simulink model "model_mussels"  (R2014b)
settings: Solver=ode45  StartTime=0.0  StopTime=40  MaxStep=0.01  RelTol=1e-3
undefined symbols (not defined in the file or in its folder): adapt, c, K, pos_0, sigma_0, speed, zeta_0
settings Model: CovSFcnEnable=on  Creator=Marta_2805  LastModifiedBy=Annie
settings SolverCC: AutoInsertRateTranBlk=on
settings OptimizationCC: UseDivisionForNetSlopeComputation=off  SimCompilerOptimization=off
settings DebuggingCC: UnderspecifiedInitializationDetection=Classic  MergeDetectMultiDrivingBlocksExec=none  FrameProcessingCompatibilityMsg=error
settings RTWCC: RTWCompilerOptimization=off

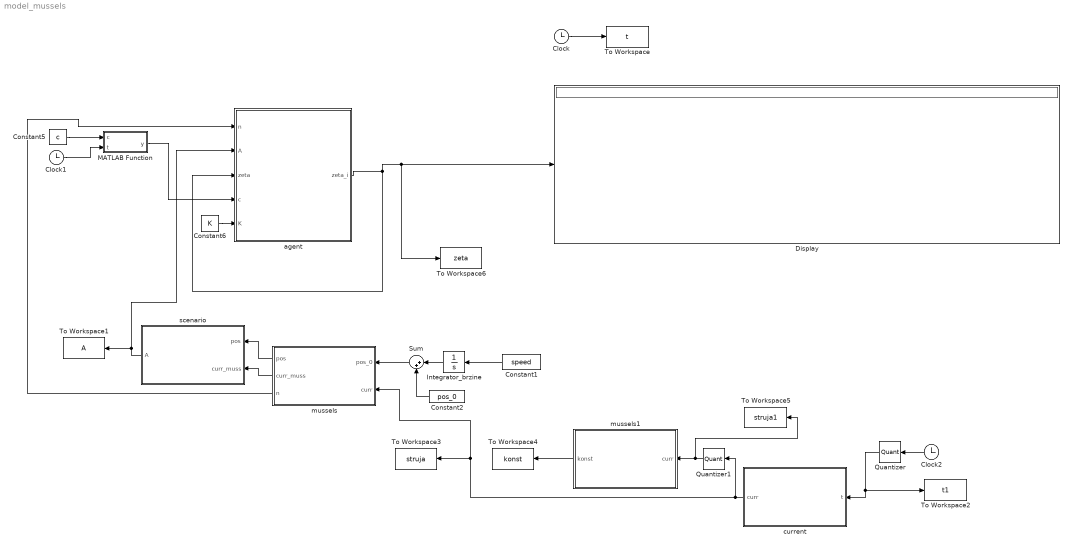
== system model_mussels ==
  Clock : Clock
  Clock1 : Clock
  Clock2 : Clock
      settings: Decimation=1000
  Constant1 : Constant  Value=speed
  Constant2 : Constant  Value=pos_0
  Constant5 : Constant  Value=c
  Constant6 : Constant  Value=K
  Display : Display
  Integrator_brzine : Integrator  InitialCondition=[0 0 0 0 0;0 0 0 0 0;0 0 0 0 0]
  MATLAB Function : MATLAB Function  TreatAsAtomicUnit=on
  Quantizer : Quantizer  QuantizationInterval=1
  Quantizer1 : Quantizer  QuantizationInterval=0.0001
  Sum : Sum  Inputs=|++
  To Workspace : ToWorkspace  VariableName=t  SampleTime=-1
  To Workspace1 : ToWorkspace  VariableName=A  SampleTime=-1
  To Workspace2 : ToWorkspace  VariableName=t1  SampleTime=-1
  To Workspace3 : ToWorkspace  VariableName=struja  SampleTime=-1
  To Workspace4 : ToWorkspace  VariableName=konst  SampleTime=-1
  To Workspace5 : ToWorkspace  VariableName=struja1  SampleTime=-1
  To Workspace6 : ToWorkspace  VariableName=zeta  SampleTime=-1
  "agent " : Subsystem
  current : MATLAB Function  TreatAsAtomicUnit=on
  mussels : MATLAB Function  TreatAsAtomicUnit=on
  mussels1 : MATLAB Function  TreatAsAtomicUnit=on
  scenario : MATLAB Function  TreatAsAtomicUnit=on
  wires:
  Constant6/1 -> "agent "/5(K)
  MATLAB Function/1(y) -> "agent "/4(c)
  "agent "/1(zeta_i) -> "agent "/3(zeta), Display/1, To Workspace6/1
  Constant5/1 -> MATLAB Function/1(c)
  Clock1/1 -> MATLAB Function/2(t)
  mussels/1(pos) -> scenario/1(pos)
  scenario/1(A) -> To Workspace1/1, "agent "/2(A)
  mussels/3(n) -> "agent "/1(n)
  Sum/1 -> mussels/1(pos_0)
  Clock/1 -> To Workspace/1
  Constant1/1 -> Integrator_brzine/1
  Constant2/1 -> Sum/2
  Integrator_brzine/1 -> Sum/1
  Clock2/1 -> Quantizer/1
  Quantizer/1 -> To Workspace2/1, current/1(t)
  current/1(curr) -> mussels/2(curr), To Workspace3/1, Quantizer1/1
  mussels/2(curr_muss) -> scenario/2(curr_muss)
  Quantizer1/1 -> mussels1/1(curr), To Workspace5/1
  mussels1/1(konst) -> To Workspace4/1

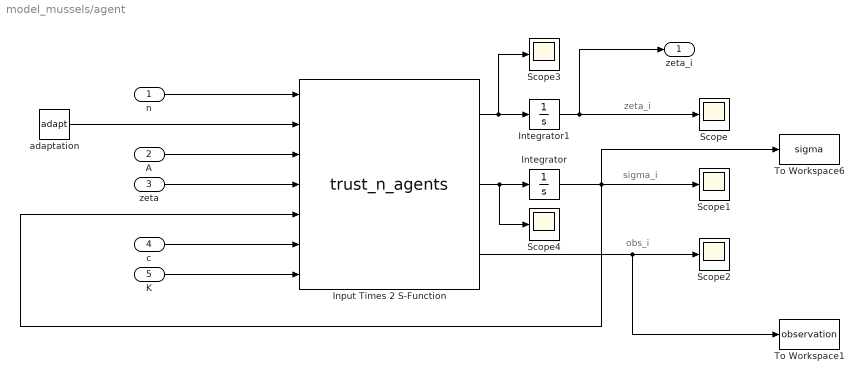
== system model_mussels/agent  ==
  note: obs_i
  note: sigma_i
  note: zeta_i
  n : Inport
  A : Inport  Port=2
  zeta : Inport  Port=3
  c : Inport  Port=4
  K : Inport  Port=5
  Input Times 2 S-Function : S-Function  FunctionName=trust_n_agents  EnableBusSupport=off
  Integrator : Integrator  InitialCondition=sigma_0
  Integrator1 : Integrator  InitialCondition=zeta_0
  Scope{,1..4} (5 alike) : Scope
      Scope settings: TimeRange=20  YMin=0.25  YMax=0.95
      Scope2 settings: YMin=0  YMax=0.2  SaveName=ScopeData2
      Scope3 settings: TimeRange=20  YMin=0.25  YMax=0.95  SaveName=ScopeData3
      Scope4 settings: TimeRange=20  YMin=0.25  YMax=0.95  SaveName=ScopeData4
  To Workspace1 : ToWorkspace  VariableName=observation  SampleTime=-1
  To Workspace6 : ToWorkspace  VariableName=sigma  SampleTime=-1
  adaptation : Constant  Value=adapt
  zeta_i : Outport
  wires:
  Integrator/1 -> Input Times 2 S-Function/5, To Workspace6/1, Scope1/1
  c/1 -> Input Times 2 S-Function/6
  K/1 -> Input Times 2 S-Function/7
  Input Times 2 S-Function/2 -> Scope4/1, Integrator/1
  Input Times 2 S-Function/1 -> Scope3/1, Integrator1/1
  Input Times 2 S-Function/3 -> To Workspace1/1, Scope2/1
  n/1 -> Input Times 2 S-Function/1
  adaptation/1 -> Input Times 2 S-Function/2
  zeta/1 -> Input Times 2 S-Function/4
  A/1 -> Input Times 2 S-Function/3
  Integrator1/1 -> zeta_i/1, Scope/1

== matlab function model_mussels/scenario ==
  data: pos input; curr_muss input; A output
function A  = scenario(pos, curr_muss)
%#codegen
%radijus komunikacije
r = 100;

n=length(pos);
%[m,n] = size(pos);
%inicijalizacija matrice A
A=zeros(n);

for i = 1:n
    for j = 1:n
        %odredivanje udaljenosti izmedju musula - prvo x, y, pa z
        distance = sqrt((pos(1,i)-pos(1,j))^2 + (pos(2,i)-pos(2,j))^2+(pos(3,i)-pos(3,j))^2);
        
        %provjera mogu li komunicirati
        if distance < r
            
            %element ne komunicira sam sa sobom
            if i == j
                A(i,j) = 0;
            else
                A(i,j) = 1;
            end
                        
        else
            A(i,j) = 0;
        end
        
    end
       
end


end

== matlab function model_mussels/mussels ==
  data: pos_0 input; pos output; curr_muss output; curr input; n output
function [pos, curr_muss, n] = mussels (pos_0, curr)
%#codegen
%u inpute bi trebalo dodati koordinate, deltu i zetu?

n=5;
pos = pos_0;

curr_ag=0;
curr_muss = zeros(n,2);
k = zeros (n,2);

X = zeros(1,n);
Y = zeros(1,n);
Z = zeros(1,n);

%mussels su blizu jedna druge

X(1) = 1;
Y(1) = 1;
Z = zeros(1,n);

for i = 2 : n
    
    X(i) = X(i-1)+0.01;
    Y(i) = Y(i-1)+0.01;

end

%mussels su rasprsene

%{
X(1) = 1;
Y(1) = 1;
Z = zeros(1,n);

for i = 2 : n
    
    X(i) = X(i-1)+10;
    Y(i) = Y(i-1)+10;

end
%}

%{
%random postavljanje koordinata
X = randperm(15,n); 
Y = randperm(15,n);
Z = zeros(1,n);
%}

%stvaranje matrice pozicije
    pos(1,:) = X;
    pos(2,:) = Y;
    pos(3,:) = Z;

%mjerenja

%agent 5 mjeri pogresnu struju
if n==5

    k = [1 1; 1 1; 1 1; 1 1; 0.5 0.5];
    curr_ag = [curr; curr; curr; curr; curr];

end

curr_muss = k.*curr_ag;

end

== matlab function model_mussels/current ==
  data: curr output; t input
function curr = current (t)
%#codegen

alfa_rad =0;
v_x=0;
v_y=0;
v = 0;

persistent brojac;
if isempty(brojac)
    brojac = 0;
end

persistent alfa;
if isempty(alfa)
    alfa = 0;
end


if t<20
    
    if mod(t, 3) == 0 & floor(t/3) > brojac
        
        brojac = brojac +1;
        alfa = alfa+3;
        
        if mod(alfa, 360) == 0
            alfa=0
        end    
    end
end

alfa_rad = alfa * pi / 180;
v=1;
v_x= v * sin(alfa_rad);
v_y= v * cos(alfa_rad);

curr=[v_x v_y];
        
end

== matlab function model_mussels/mussels1 ==
  data: konst output; curr input
function konst = comparison (curr)
%#codegen

konst=0;
threshold = 1e-5; 

%curr
wanted =[0.1564, 0.9877];


if all(abs(wanted - curr)<= threshold)
 
       konst = 1
  
end

end

== matlab function model_mussels/MATLAB Function ==
  data: c input; y output; t input
function y = fcn(c, t)
%#codegen
if t > 25
    c(:,1) = c(:,1);
%    c(:,13) = c(:,13) / 5; 
%    c(:,13) = c(:,13) / 7;
%    c(:,3) = c(:,3) * 2;
end
y = c;
